simulink model "Li_ion_model"  (R2020a)
settings: Solver=VariableStepAuto  StartTime=0.0  StopTime=1180  MaxStep=0.001  RelTol=1e-3
values from neighbouring files (symbols this model uses):
  C1_LUT = [1913.6,12447,30609 ... (first row only)    [Cell_Script.m]
  Capacity_LUT = [28.01,27.63,27.64]    [Cell_Script.m]
  cell_area = cell_length*cell_width    (= 0.051302)    [Cell_Script.m]
  cell_Cp_heat = 810.5328    [Cell_Script.m]
  cell_mass = 0.720    (= 0.72)    [Cell_Script.m]
  Em_LUT = [3.49,3.51,3.52;3.55,3.56,3.56 ... (first row only)    [Cell_Script.m]
  h_conv = 5    [Cell_Script.m]
  R0_LUT = [0.0117,0.0085,0.0090;0.0110,0.0085,0.0090 ... (first row only)    [Cell_Script.m]
  R1_LUT = [0.0109,0.0029,0.0013;0.0069,0.0024,0.0012 ... (first row only)    [Cell_Script.m]
  SOC_LUT = [0;0.100;0.250;0.500;0.750;0.900;1.00]    [Cell_Script.m]
  T_init = 293.15    [Cell_Script.m]
  Temperature_LUT = [278.15,293.15,313.15]    [Cell_Script.m]
settings Model: Creator=shaurya  LastModifiedBy=shaurya

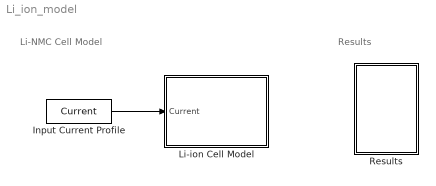
== system Li_ion_model ==
  note: Results
  note: Li-NMC Cell Model
  Input Current Profile : FromWorkspace  VariableName=Current
  Li-ion Cell Model : Subsystem
  Results : Subsystem
  wires:
  Input Current Profile/1 -> Li-ion Cell Model/1(Current)

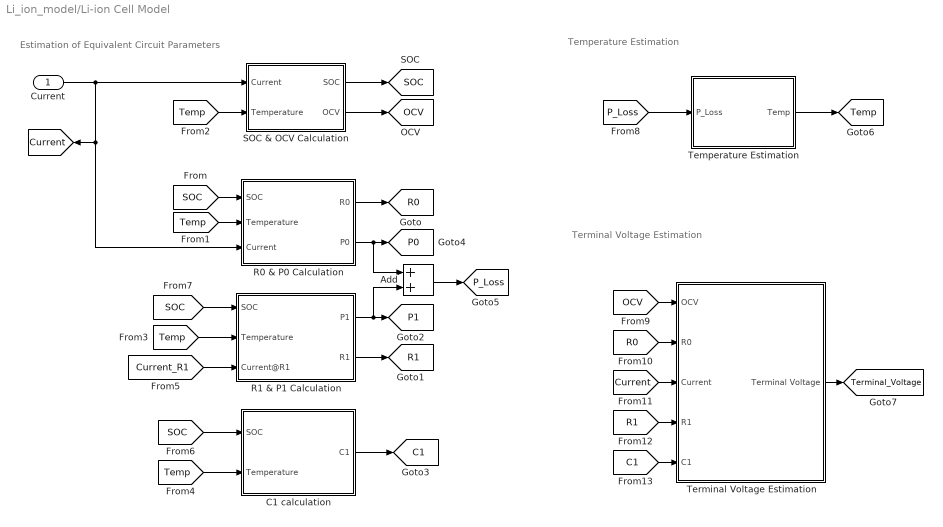
== system Li_ion_model/Li-ion Cell Model ==
  note: Terminal Voltage Estimation
  note: Temperature Estimation
  note: Estimation of Equivalent Circuit Parameters
  Current : Inport
  Add : Sum
  C1 calculation : Subsystem
  R0 & P0 Calculation : Subsystem
  R1 & P1 Calculation : Subsystem
  SOC & OCV Calculation : Subsystem
  Temperature Estimation : Subsystem
  Terminal Voltage Estimation : Subsystem
  tag scope: C1=global, Current=global, OCV=global, P0=global, P1=global, P_Loss=global, R0=global, R1=global, SOC=global, Temp=global, Terminal_Voltage=global
  wires:
  Current/1 -> R0 & P0 Calculation/3(Current), [Current], SOC & OCV Calculation/1(Current)
  R0 & P0 Calculation/1(R0) -> [R0]
  SOC & OCV Calculation/1(SOC) -> [SOC]
  [SOC] -> R0 & P0 Calculation/1(SOC)
  SOC & OCV Calculation/2(OCV) -> [OCV]
  C1 calculation/1(C1) -> [C1]
  R1 & P1 Calculation/1(P1) -> Add/2, [P1]
  R1 & P1 Calculation/2(R1) -> [R1]
  R0 & P0 Calculation/2(P0) -> Add/1, [P0]
  [Temp] -> R0 & P0 Calculation/2(Temperature)
  [Temp] -> R1 & P1 Calculation/2(Temperature)
  [Temp] -> SOC & OCV Calculation/2(Temperature)
  [Temp] -> C1 calculation/2(Temperature)
  [Current_R1] -> R1 & P1 Calculation/3(Current@R1)
  [SOC] -> C1 calculation/1(SOC)
  [SOC] -> R1 & P1 Calculation/1(SOC)
  Add/1 -> [P_Loss]
  Temperature Estimation/1(Temp) -> [Temp]
  [P_Loss] -> Temperature Estimation/1(P_Loss)
  Terminal Voltage Estimation/1(Terminal Voltage) -> [Terminal_Voltage]
  [OCV] -> Terminal Voltage Estimation/1(OCV)
  [R0] -> Terminal Voltage Estimation/2(R0)
  [Current] -> Terminal Voltage Estimation/3(Current)
  [R1] -> Terminal Voltage Estimation/4(R1)
  [C1] -> Terminal Voltage Estimation/5(C1)

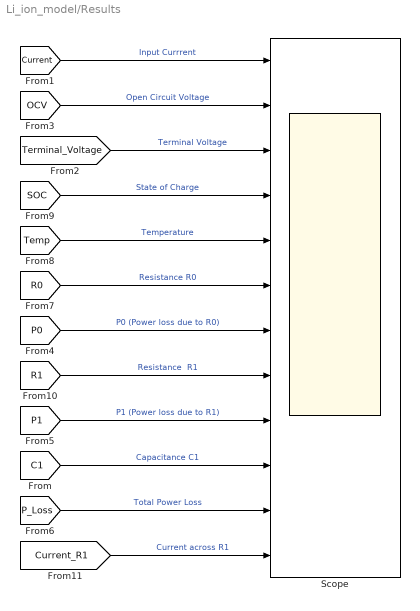
== system Li_ion_model/Results ==
  "Scope " : Scope  NumInputPorts=12
  wires:
  [Current] -> "Scope "/1  "Input Currrent"
  [OCV] -> "Scope "/2  "Open Circuit Voltage"
  [SOC] -> "Scope "/4  "State of Charge"
  [Terminal_Voltage] -> "Scope "/3  "Terminal Voltage"
  [Temp] -> "Scope "/5  "Temperature"
  [R0] -> "Scope "/6  "Resistance R0"
  [P0] -> "Scope "/7  "P0 (Power loss due to R0)"
  [R1] -> "Scope "/8  "Resistance  R1"
  [P1] -> "Scope "/9  "P1 (Power loss due to R1)"
  [C1] -> "Scope "/10  "Capacitance C1"
  [P_Loss] -> "Scope "/11  "Total Power Loss"
  [Current_R1] -> "Scope "/12  "Current across R1"

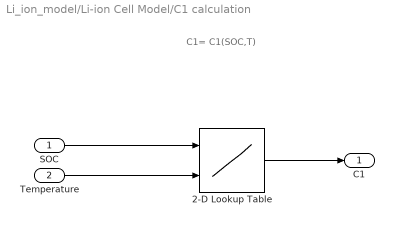
== system Li_ion_model/Li-ion Cell Model/C1 calculation ==
  note: C1= C1(SOC,T)
  SOC : Inport
  Temperature : Inport  Port=2
  2-D Lookup Table : Lookup_n-D  BreakpointsForDimension1=SOC_LUT  BreakpointsForDimension2=Temperature_LUT  Table=C1_LUT  InternalRulePriority=Speed  RndMeth=Simplest  InputSameDT=on
  C1 : Outport
  wires:
  2-D Lookup Table/1 -> C1/1
  Temperature/1 -> 2-D Lookup Table/2
  SOC/1 -> 2-D Lookup Table/1

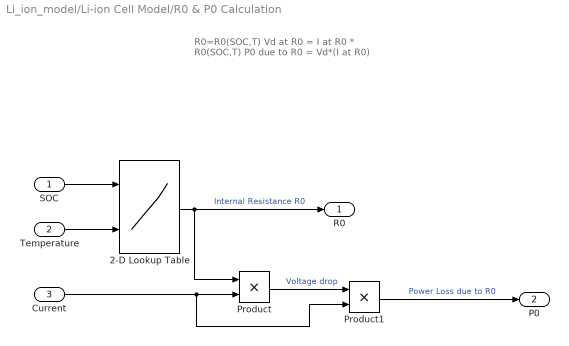
== system Li_ion_model/Li-ion Cell Model/R0 & P0 Calculation ==
  note: R0=R0(SOC,T)
      | Vd at R0 = I at R0 * R0(SOC,T)
      | P0 due to R0 = Vd*(I at R0)
  SOC : Inport
  Temperature : Inport  Port=2
  Current : Inport  Port=3
  2-D Lookup Table : Lookup_n-D  BreakpointsForDimension1=SOC_LUT  BreakpointsForDimension2=Temperature_LUT  Table=R0_LUT  InternalRulePriority=Speed  RndMeth=Simplest  InputSameDT=on
  Product : Product
  Product1 : Product
  R0 : Outport
  P0 : Outport  Port=2
  wires:
  SOC/1 -> 2-D Lookup Table/1
  Temperature/1 -> 2-D Lookup Table/2
  2-D Lookup Table/1 -> Product/1, R0/1  "Internal Resistance R0"
  Current/1 -> Product1/2, Product/2
  Product/1 -> Product1/1  "Voltage drop"
  Product1/1 -> P0/1  "Power Loss due to R0"

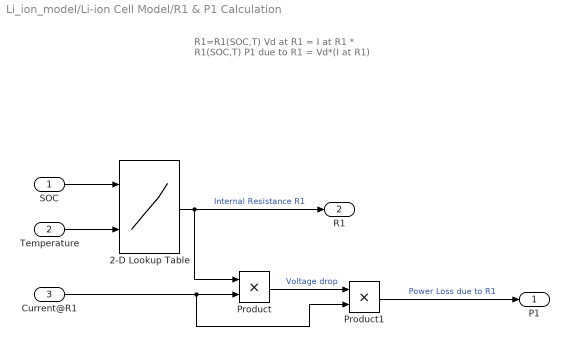
== system Li_ion_model/Li-ion Cell Model/R1 & P1 Calculation ==
  note: R1=R1(SOC,T)
      | Vd at R1 = I at R1 * R1(SOC,T)
      | P1 due to R1 = Vd*(I at R1)
  SOC : Inport
  Temperature : Inport  Port=2
  Current@R1 : Inport  Port=3
  2-D Lookup Table : Lookup_n-D  BreakpointsForDimension1=SOC_LUT  BreakpointsForDimension2=Temperature_LUT  Table=R1_LUT  InternalRulePriority=Speed  RndMeth=Simplest  InputSameDT=on
  Product : Product
  Product1 : Product
  P1 : Outport
  R1 : Outport  Port=2
  wires:
  SOC/1 -> 2-D Lookup Table/1
  Temperature/1 -> 2-D Lookup Table/2
  2-D Lookup Table/1 -> Product/1, R1/1  "Internal Resistance R1"
  Current@R1/1 -> Product1/2, Product/2
  Product/1 -> Product1/1  "Voltage drop"
  Product1/1 -> P1/1  "Power Loss due to R1"

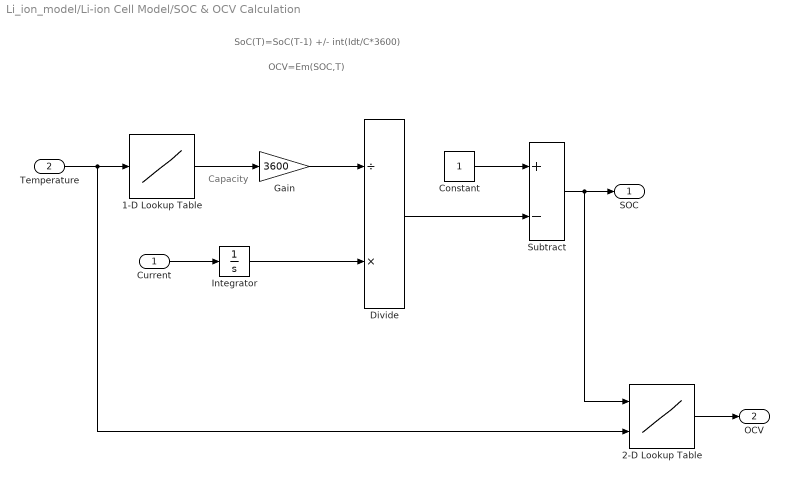
== system Li_ion_model/Li-ion Cell Model/SOC & OCV Calculation ==
  note: OCV=Em(SOC,T)
  note: Capacity
  note: SoC(T)=SoC(T-1) +/- int(Idt/C*3600)
  Current : Inport
  Temperature : Inport  Port=2
  1-D Lookup Table : Lookup_n-D  NumberOfTableDimensions=1  BreakpointsForDimension1=Temperature_LUT  Table=Capacity_LUT  InternalRulePriority=Speed  RndMeth=Simplest  InputSameDT=on
  2-D Lookup Table : Lookup_n-D  BreakpointsForDimension1=SOC_LUT  BreakpointsForDimension2=Temperature_LUT  Table=Em_LUT  InternalRulePriority=Speed  RndMeth=Simplest  InputSameDT=on
  Constant : Constant
  Divide : Product  Inputs=/*
  Gain : Gain  Gain=3600
  Integrator : Integrator
  Subtract : Sum  Inputs=+-
  SOC : Outport
  OCV : Outport  Port=2
  wires:
  Temperature/1 -> 2-D Lookup Table/2, 1-D Lookup Table/1
  1-D Lookup Table/1 -> Gain/1
  Current/1 -> Integrator/1
  Gain/1 -> Divide/1
  Integrator/1 -> Divide/2
  Constant/1 -> Subtract/1
  Divide/1 -> Subtract/2
  Subtract/1 -> 2-D Lookup Table/1, SOC/1
  2-D Lookup Table/1 -> OCV/1

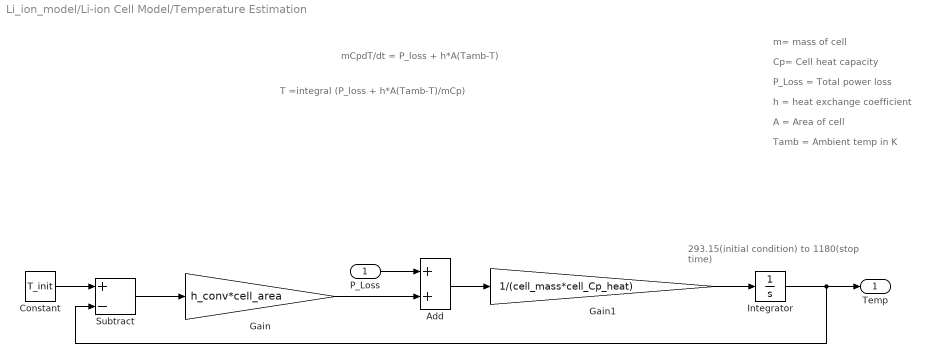
== system Li_ion_model/Li-ion Cell Model/Temperature Estimation ==
  note: 293.15(initial condition) to 1180(stop time)
  note: T =integral (P_loss + h*A(Tamb-T)/mCp)
  note: Tamb = Ambient temp in K
  note: A = Area of cell
  note: h = heat exchange coefficient
  note: P_Loss = Total power loss
  note: Cp= Cell heat capacity
  note: m= mass of cell
  note: mCpdT/dt = P_loss + h*A(Tamb-T)
  P_Loss : Inport
  Add : Sum
  Constant : Constant  Value=T_init
  Gain : Gain  Gain=h_conv*cell_area
  Gain1 : Gain  Gain=1/(cell_mass*cell_Cp_heat)
  Integrator : Integrator  InitialCondition=293.15
  Subtract : Sum  Inputs=+-
  Temp : Outport
  wires:
  Constant/1 -> Subtract/1
  Subtract/1 -> Gain/1
  Gain/1 -> Add/2
  P_Loss/1 -> Add/1
  Add/1 -> Gain1/1
  Gain1/1 -> Integrator/1
  Integrator/1 -> Subtract/2, Temp/1

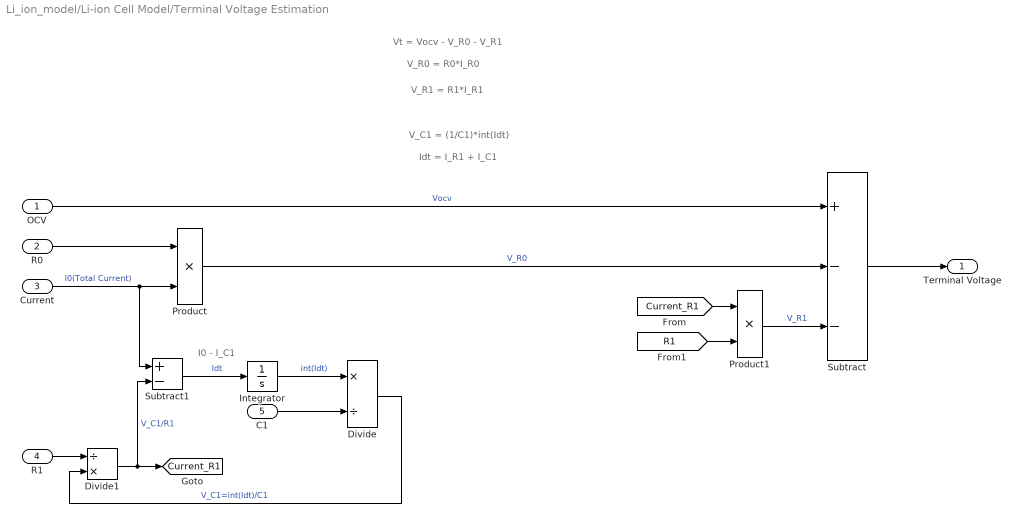
== system Li_ion_model/Li-ion Cell Model/Terminal Voltage Estimation ==
  note: I0 - I_C1
  note: Idt = I_R1 + I_C1
  note: V_C1 = (1/C1)*int(Idt)
  note: V_R1 = R1*I_R1
  note: V_R0 = R0*I_R0
  note: Vt = Vocv - V_R0 - V_R1
  OCV : Inport
  R0 : Inport  Port=2
  Current : Inport  Port=3
  R1 : Inport  Port=4
  C1 : Inport  Port=5
  Divide : Product  Inputs=*/
  Divide1 : Product  Inputs=/*
  Integrator : Integrator
  Product : Product
  Product1 : Product
  Subtract : Sum  Inputs=+--
  Subtract1 : Sum  Inputs=+-
  Terminal Voltage : Outport
  tag scope: Current_R1=global
  wires:
  OCV/1 -> Subtract/1  "Vocv"
  R0/1 -> Product/1
  Current/1 -> Subtract1/1, Product/2  "I0(Total Current)"
  Product/1 -> Subtract/2  "V_R0"
  Product1/1 -> Subtract/3  "V_R1"
  [Current_R1] -> Product1/1
  [R1] -> Product1/2
  Integrator/1 -> Divide/1  "int(Idt)"
  C1/1 -> Divide/2
  R1/1 -> Divide1/1
  Divide/1 -> Divide1/2  "V_C1=int(Idt)/C1"
  Divide1/1 -> Subtract1/2, [Current_R1]  "V_C1/R1"
  Subtract1/1 -> Integrator/1  "Idt"
  Subtract/1 -> Terminal Voltage/1
